simulink library "PaPI"  (R2014b)
settings: Solver=ode45  StartTime=0.0  StopTime=10.0  RelTol=1e-3
undefined symbols (not defined in the file or in its folder): unicode2native
libraries: PaPI x2
settings Model: Creator=sven  LastModifiedBy=sven

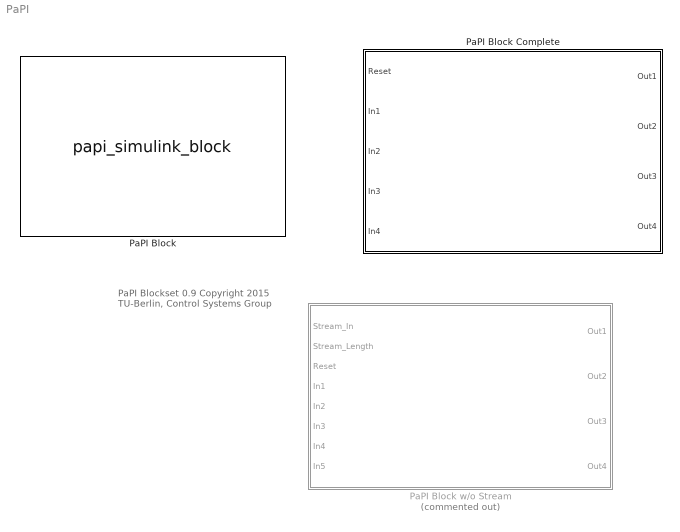
== system PaPI ==
  note: PaPI Blockset 0.9
      | Copyright 2015
      | TU-Berlin, Control Systems Group
  PaPI Block : S-Function  FunctionName=papi_simulink_block  Parameters=amount_parameters, [unicode2native(json_string, 'ISO-8859-1') 0], output_size, sum(amount_parameters), define_inputs, split_inputs, UDPLocalPort, UDPRemotePort, [unicode2native(UDPRemoteIP, 'ISO-8859-1') 0], UDPStart  EnableBusSupport=off  mask(PaPI Block){amount_parameters=[1,2,3,4,5], split_inputs=[1,1,1,1,1], define_inputs=[1,2,3,4,5], json_string='{}', output_size=200, sum_parameters=5, UDPLocalPort=20001, UDPRemotePort=20000, UDPRemoteIP='127.0.0.1', UDPStart=on}
      mask prompts: split_inputs "Split input signals"; define_inputs "Define input signals"; sum_parameters "Sum parameters"; UDPLocalPort "UDP Local Port"; UDPRemotePort "UDP Remote Port"; UDPRemoteIP "UDP Remote IP"; UDPStart "UDP Handle start"
      mask help: Basic Block for the communication of Simulink <-> PaPI
      mask Help:
      | Take a look here:
      | 
      | https://github.com/TUB-Control/PaPI/wiki
      mask Display:
      | port_label('input',1,'Data');
      | port_label('input',2,'SimTime');
      | port_label('input',3,'Control');
      | 
      | port_label('output',1,'Parameter');
  PaPI Block Complete : Subsystem  mask(PaPI Block Complete){amount_parameters=[1,2,3,4], define_inputs=[1,1,1,1], split_inputs=[1,1,1,1], json_string='{}', UDPLocalPort=20001, UDPRemotePort=20000, UDPRemoteIP='127.0.0.1', output_size=200, UDPStart=on, sample_time=-1}
      mask prompts: amount_parameters "Amount parameters"; define_inputs "Define input signals"; split_inputs "Split input signals"; json_string "Json Config"; UDPLocalPort "UDP Local Port"; UDPRemotePort "UDP Remote Port"; UDPRemoteIP "UDP Remote IP"; output_size "Output size"; UDPStart "UDP Handle start"; sample_time "Sampling Rate"
      mask help:
      | The UDP communication is realized by the boost library.
      | More dynamic behavior by defining inputs (signals) and outputs (parameters).
      mask init:
      | papi_block_complete_init(gcb, amount_parameters, size(define_inputs,2) , json_string, define_inputs, split_inputs)
      mask Help:
      | <p><a href="https://github.com/TUB-Control/PaPI/wiki">https://github.com/TUB-Control/PaPI/wiki</a></p>
      | 
      | <h4>This blocks provides following static input signal</h4>
      | 
      | <b>reset</b>: Possible values {0,1}
      | This signal can be used to reset the PaPI Block. The Configuration will be sent again and the current outputs will be to zero.
      | </hr>
      | <h4>This blocks provides following parameters</h4>
      | 
      | <b>[Amount parameters]</b>
      | Used to define the parameters which can be modified in PaPI.
      | [1,2,45] creates two parameters, with size(p1)=1, size(p2)=2, size(p3)=45
      | 
      | <b>[Json Config]</b>
      | Can be used to create Plugins and subcriptions in PaPI.
      | 
      | <b>[Amount of signals]</b>
      | Defines the amount of input signals which can be subscribed in PaPI
      | 
      | <b>[Local port]</b>
      | <b>[Remote port]</b>
      | <b>[Output size]</b>
      | Defines the maximal vector size which can be sent at a single timestamp.
      | 
      | <b>[Recieve: Msg Length]</b>
      | Defines the maximal vector size which can be recieved at a single timestamp.
      | 
      | <b>[Local IP]</b>
      | <b>[Remote IP]</b>
      mask TypeOptions amount_parameters: PaPI Block/amount_parameters
      mask TypeOptions define_inputs: PaPI Block/define_inputs
      mask TypeOptions split_inputs: PaPI Block/split_inputs
      mask TypeOptions UDPLocalPort: PaPI Block/UDPLocalPort
      mask TypeOptions UDPRemotePort: PaPI Block/UDPRemotePort
      mask TypeOptions UDPRemoteIP: PaPI Block/UDPRemoteIP
      mask TypeOptions output_size: PaPI Block/output_size
      mask TypeOptions UDPStart: PaPI Block/UDPStart
      mask TypeOptions sample_time: Digital Clock/SampleTime
      mask Display: port_label('input',  1  ,' Control ');port_label('input', 2 ,'s1');port_label('input', 3 ,'s2');port_label('input', 4 ,'s3');port_label('input', 5 ,'s4'); port_label('output',  1  ,' p1 '); port_label('output',  2  ,' p2 '); port_label('output',  3  ,' p3 '); port_label('output',  4  ,' p4 ');
  PaPI Block w/o Stream : Subsystem  Commented=on  mask(PaPI Block w/o Stream){amount_parameters=[1,2,3,4], define_inputs=[1,1,1,2,3], split_signals=[1,1,1,1,1], json_string='{}', sample_time=1, output_size=200}
      mask prompts: amount_parameters "Amount parameters"; define_inputs "Define input signals"; split_signals "Split input signals"; json_string "Json Config"; sample_time "Sampling Rate"; output_size "Output size"
      mask help:
      | Stream source and target is missing, e.g. a UDP stream.
      | More dynamic behavior by defining inputs (signals) and outputs (parameters).
      mask init:
      | papi_block_wo_stream_init( gcb, amount_parameters, size(define_inputs,2), json_string, define_inputs, split_signals)
      mask Help:
      | Take a look here:
      | 
      | https://github.com/TUB-Control/PaPI/wiki
      | 
      | Signals -----------------------------
      | 
      | 'Stream_In': Input stream from PaPI
      | 'Stream_Out': Output stream from PaPI
      | 
      | 'Stream_Length': Current new message length.
      | 
      | 'reset'==0: Configuration will be sent again, sets current outputs to zero.
      | 
      | Parameters -----------------------------
      | 
      | Amount parameters :
      | Used to define the parameters which can be modified in PaPI.
      | [1,2,45] creates two parameters, with size(p1)=1, size(p2)=2, size(p3)=45
      | 
      | Json Config:
      | Can be used to create Plugins and subcriptions in PaPI.
      | 
      | Amount of signals:
      | Defines the amount of input signals which can be subscribed in PaPI
      | 
      | Output size:
      | Defines the maximal size which can be sent at a single timestamp.
      mask TypeOptions amount_parameters: PaPI Block/amount_parameters
      mask TypeOptions define_inputs: PaPI Block/define_inputs
      mask TypeOptions split_signals: PaPI Block/split_inputs
      mask TypeOptions sample_time: Digital Clock/SampleTime
      mask Display: port_label('input',  1  ,' Stream_In ');port_label('input',  2  ,' Stream_length ');port_label('input',  3  ,' Reset ');port_label('output',  1  ,' Stream_out ');port_label('input', 4 ,'s1');port_label('input', 5 ,'s2');port_label('input', 6 ,'s3');port_label('input', 7 ,'s4');port_label('input', 8 ,'s5'); port_label('output',  2  ,' p1 '); port_label('output',  3  ,' p2 '); port_label('output',  4  ,' p3 ');

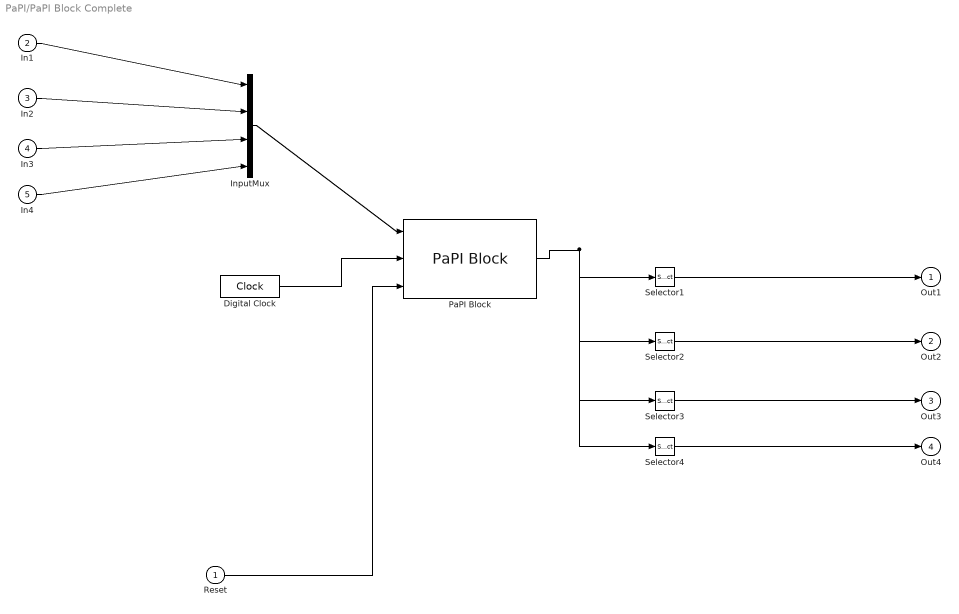
== system PaPI/PaPI Block Complete ==
  Reset : Inport  PortDimensions=1
  In1 : Inport  Port=2  PortDimensions=1
  In2 : Inport  Port=3  PortDimensions=1
  In3 : Inport  Port=4  PortDimensions=1
  In4 : Inport  Port=5  PortDimensions=1
  Digital Clock : DigitalClock  SampleTime=sample_time
  InputMux : Mux
  PaPI Block : PaPI/PaPI Block  amount_parameters=amount_parameters  split_inputs=split_inputs  define_inputs=define_inputs  json_string="'{\"BlockConfig\": {\"ParameterNames\": [\"p1\",\"p2\",\"p3\",\"p4\"],\"SignalNames\": [\"s1\",\"s2\",\"s3\",\"s4\"]}}'"  output_size=output_size  sum_parameters=5  UDPLocalPort=UDPLocalPort  UDPRemotePort=UDPRemotePort  UDPRemoteIP=UDPRemoteIP  UDPStart=on
  Selector1 : Selector  InputPortWidth=10  Indices=[1:1]
  Selector2 : Selector  InputPortWidth=10  Indices=[2:3]
  Selector3 : Selector  InputPortWidth=10  Indices=[4:6]
  Selector4 : Selector  InputPortWidth=10  Indices=[7:10]
  Out1 : Outport
  Out2 : Outport  Port=2
  Out3 : Outport  Port=3
  Out4 : Outport  Port=4
  wires:
  Digital Clock/1 -> PaPI Block/2
  Selector1/1 -> Out1/1
  Selector2/1 -> Out2/1
  Selector3/1 -> Out3/1
  Selector4/1 -> Out4/1
  PaPI Block/1 -> Selector1/1, Selector2/1, Selector3/1, Selector4/1
  Reset/1 -> PaPI Block/3
  InputMux/1 -> PaPI Block/1
  In1/1 -> InputMux/1
  In2/1 -> InputMux/2
  In3/1 -> InputMux/3
  In4/1 -> InputMux/4

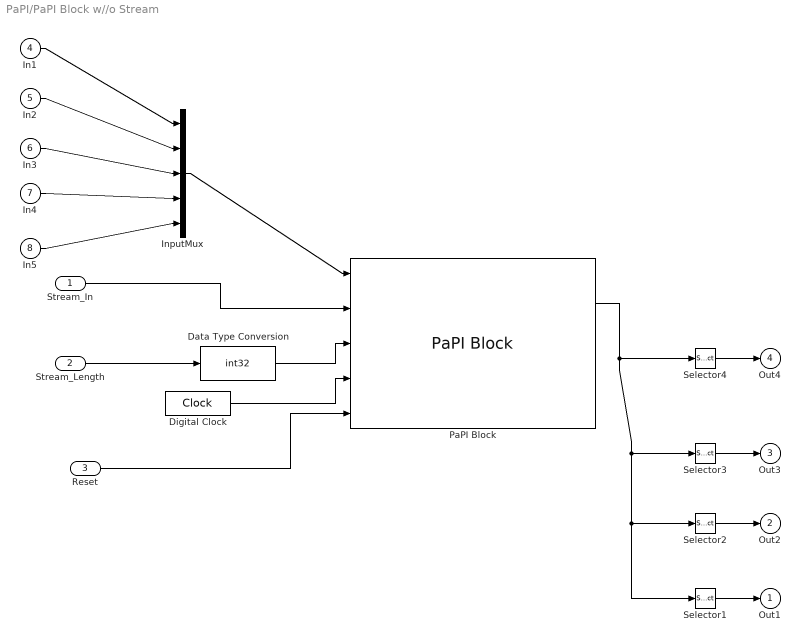
== system PaPI/PaPI Block w//o Stream ==
  Stream_In : Inport
  Stream_Length : Inport  Port=2
  Reset : Inport  Port=3
  In1 : Inport  Port=4  PortDimensions=1
  In2 : Inport  Port=5  PortDimensions=1
  In3 : Inport  Port=6  PortDimensions=1
  In4 : Inport  Port=7  PortDimensions=2
  In5 : Inport  Port=8  PortDimensions=3
  Data Type Conversion : DataTypeConversion  OutDataTypeStr=int32
  Digital Clock : DigitalClock  SampleTime=sample_time
  InputMux : Mux  Inputs=5
  PaPI Block : PaPI/PaPI Block  amount_parameters=amount_parameters  split_inputs=split_signals  define_inputs=define_inputs  json_string="'{\"BlockConfig\": {\"ParameterNames\": [\"p1\",\"p2\",\"p3\"],\"SignalNames\": [\"s1\",\"s2\",\"s3\",\"s4(1)\",\"s4(2)\",\"s5(1)\",\"s5(2)\",\"s5(3)\"]}}'"  output_size=200  sum_parameters=5  UDPLocalPort=0  UDPRemotePort=0  UDPRemoteIP=0
  Selector1 : Selector  InputPortWidth=10  Indices=[1:1]
  Selector2 : Selector  InputPortWidth=10  Indices=[2:3]
  Selector3 : Selector  InputPortWidth=10  Indices=[4:6]
  Selector4 : Selector  InputPortWidth=10  Indices=[7:10]
  Out1 : Outport
  Out2 : Outport  Port=2
  Out3 : Outport  Port=3
  Out4 : Outport  Port=4
  wires:
  Digital Clock/1 -> PaPI Block/4
  Stream_Length/1 -> Data Type Conversion/1
  Stream_In/1 -> PaPI Block/2
  Data Type Conversion/1 -> PaPI Block/3
  Reset/1 -> PaPI Block/5
  Selector1/1 -> Out1/1
  PaPI Block/1 -> Selector1/1, Selector2/1, Selector3/1, Selector4/1
  Selector2/1 -> Out2/1
  Selector3/1 -> Out3/1
  Selector4/1 -> Out4/1
  InputMux/1 -> PaPI Block/1
  In1/1 -> InputMux/1
  In2/1 -> InputMux/2
  In3/1 -> InputMux/3
  In4/1 -> InputMux/4
  In5/1 -> InputMux/5
